simulink model "Green_H2_Battery_Solar"  (R2025a)
settings: Solver=FixedStepAuto  StartTime=0.0  StopTime=24*3600*7  FixedStep=Ts_Control  MaxStep=0.1  RelTol=1e-3  AbsTol=1e-3
values from neighbouring files (symbols this model uses):
  R_h2 = 4.12    [Hydrogen_Prop_File.m]
  Ts = 10    [Parameter_File.m]
undefined symbols (not defined in the file or in its folder): Battery, DiscIntNeverNeededParam, Electric, Operation_Ref, Plate
libraries: fl_lib x25, nesl_utility x20, ee_lib x3, simulink x2, batteryecm_lib x1
(part 4 of 4)

== matlab function Green_H2_Battery_Solar/Solar Array/MPPT/MPPT Controller using Perturb & Observe technique  ==
  settings: updateMethod=DISCRETE  sampleTime=Ts_Control
  data: Param input; Enabled input; V input; I input; D output
function D  = PandO(Param, Enabled, V, I)

% MPPT controller based on the Perturb & Observe algorithm.

% D output = Duty cycle of the boost converter (value between 0 and 1)
%
% Enabled input = 1 to enable the MPPT controller
% V input = PV array terminal voltage (V)
% I input = PV array current (A)
%
% Param input:
Dinit = Param(1);  %Initial value for D output
Dmax = Param(2);   %Maximum value for D
Dmin = Param(3);   %Minimum value for D
deltaD = Param(4); %Increment value used to increase/decrease the duty cycle D
% ( increasing D = decreasing Vref )
%  

persistent Vold Pold Dold;

dataType = 'double';

if isempty(Vold)
    Vold=0;
    Pold=0;
    Dold=Dinit;
end
P= V*I;
dV= V - Vold;
dP= P - Pold;

 if dP ~= 0 & Enabled ~=0
%     if dP>1e-9  & dP<-1e-9 & Enabled ~=0
    if dP < 0
        if dV < 0
            D = Dold - deltaD;
        else
            D = Dold + deltaD;
        end
    else
        if dV < 0
            D = Dold + deltaD;
        else
            D = Dold - deltaD;
        end    
    end
else D=Dold;
end

if D >= Dmax | D<= Dmin
    D=Dold;
end

Dold=D;
Vold=V;
Pold=P;

== matlab function Green_H2_Battery_Solar/Energy Storage (Battery)/Iref = f(I_solar, Qbat) ==
  data: u input; y output; u1 input; y1 input; f input
function y = fcn(u, u1, y1, f)

y = interp1(u1, f*y1, u, 'linear', 'extrap');
